simulink model "Lorenz_system"  (R2021a)
settings: Solver=ode45  StartTime=0  StopTime=1/10  RelTol=1e-3
model workspace (MAT data in the model file):
  Beta = 2.66666666667
  Rho = 28
  Sigma = 10
  X0 = Simulink.Parameter
  X0.Value = 10
  X0.DataType = 'auto'
  X0.Dimensions = [1 1]
  Y0 = Simulink.Parameter
  Y0.Value = 20
  Y0.DataType = 'auto'
  Y0.Dimensions = [1 1]
  Z0 = Simulink.Parameter
  Z0.Value = 10
  Z0.DataType = 'auto'
  Z0.Dimensions = [1 1]
settings Model: OrderedModelArguments=off  Creator=The MathWorks, Inc.  LastModifiedBy=The MathWorks, Inc.

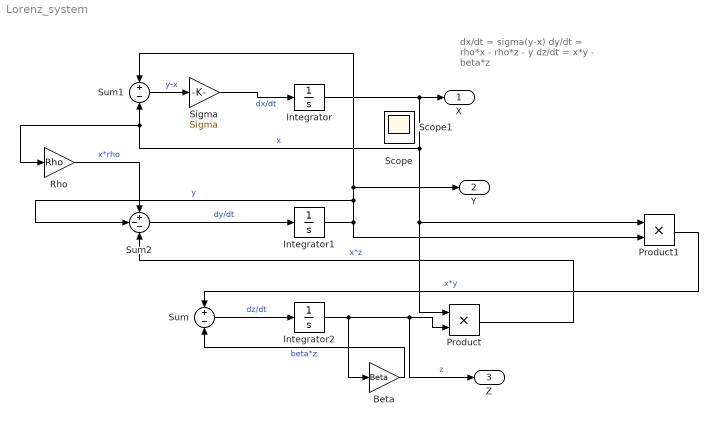
== system Lorenz_system ==
  note: dx/dt = sigma(y-x)
      | dy/dt = rho*x - rho*z - y
      | dz/dt = x*y - beta*z
  Beta : Gain  Gain=Beta
  Integrator : Integrator  InitialCondition=X0  ContinuousStateAttributes='x'
  Integrator1 : Integrator  InitialCondition=Y0  ContinuousStateAttributes='y'
  Integrator2 : Integrator  InitialCondition=Z0  ContinuousStateAttributes='z'
  Product : Product
  Product1 : Product
  Rho : Gain  Gain=Rho
  Sigma : Gain  Gain=Sigma
  Sum : Sum  Inputs=+-
  Sum1 : Sum  Inputs=+-
  Sum2 : Sum  Inputs=+--
  X : Outport
  Y : Outport  Port=2
  Z : Outport  Port=3
  Scope : Scope
  Scope1 : Scope
  wires:
  Integrator/1 -> X/1, Product1/1, Product/1, Rho/1, Sum1/2  "x"
  Integrator1/1 -> Sum2/2, Y/1, Sum1/1, Product1/2  "y"
  Sum1/1 -> Sigma/1  "y-x"
  Sigma/1 -> Integrator/1  "dx/dt"
  Sum2/1 -> Integrator1/1  "dy/dt"
  Rho/1 -> Sum2/1  "x*rho"
  Integrator2/1 -> Beta/1, Z/1, Product/2  "z"
  Product/1 -> Sum2/3  "x*z"
  Product1/1 -> Sum/1  "x*y"
  Beta/1 -> Sum/2  "beta*z"
  Sum/1 -> Integrator2/1  "dz/dt"
